simulink model "reto4_simu"  (R2024a)
settings: Solver=FixedStepAuto  StartTime=0.0  StopTime=20.0  FixedStep=0.0001  RelTol=1e-3
libraries: cstblocks x2, simulink x1
settings Model: Creator=Usuario  LastModifiedBy=Usuario

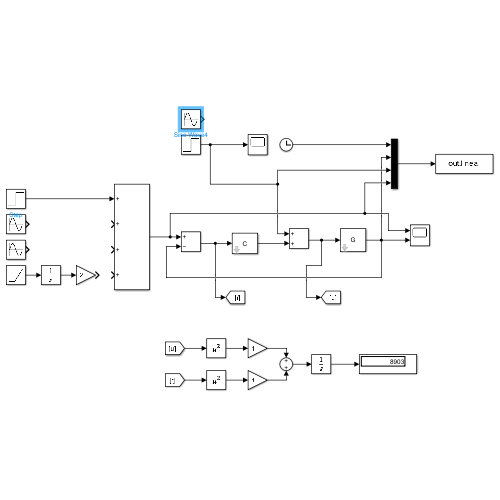
[thumbnail: Simulink's stored preview of the top-level diagram]
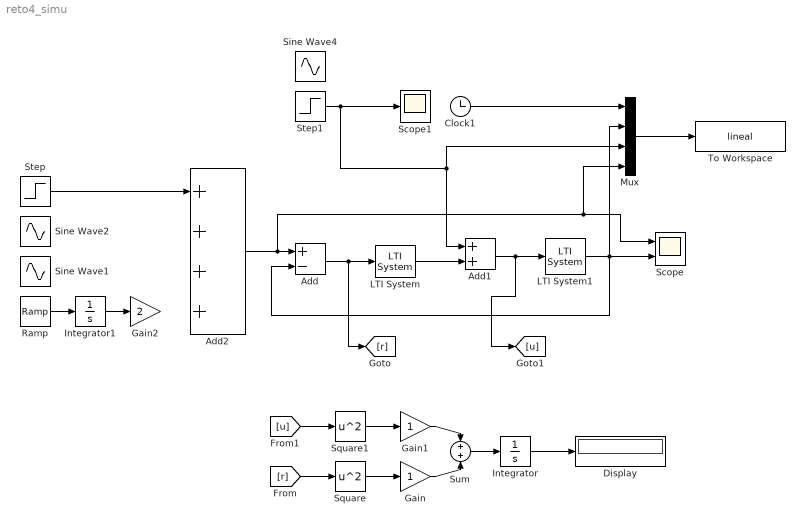
== system reto4_simu ==
  Add : Sum  Inputs=+-
  Add1 : Sum
  Add2 : Sum  Inputs=++++
  Clock1 : Clock
  Display : Display
  Gain : Gain
  Gain1 : Gain
  Gain2 : Gain  Gain=2
  Integrator : Integrator
  Integrator1 : Integrator
  LTI System : cstblocks/LTI System  sys=C  IC=[]  PadeOrder=0
  LTI System1 : cstblocks/LTI System  sys=G  IC=[]  PadeOrder=0
  Mux : Mux
  Ramp : simulink/Sources/Ramp  slope=1  start=0  InitialOutput=0
  Scope : Scope  NumInputPorts=2
  Scope1 : Scope
  Sine Wave1 : Sin  Frequency=2  Phase=pi/2+6  SampleTime=0
  Sine Wave2 : Sin  Frequency=2  SampleTime=0
  Sine Wave4 : Sin  Phase=pi  SampleTime=0
  Square : Math  Operator=square
  Square1 : Math  Operator=square
  Step : Step  Time=0  After=2  SampleTime=0
  Step1 : Step  Time=0  After=50  SampleTime=0
  Sum : Sum
  To Workspace : ToWorkspace  VariableName=lineal  SampleTime=-1
  wires:
  LTI System1/1 -> Mux/2, Scope/2, Add/2
  Add1/1 -> [u], LTI System1/1
  LTI System/1 -> Add1/2
  Add/1 -> [r], LTI System/1
  Add2/1 -> Mux/4, Scope/1, Add/1
  [r] -> Square/1
  [u] -> Square1/1
  Square/1 -> Gain/1
  Square1/1 -> Gain1/1
  Gain1/1 -> Sum/1
  Gain/1 -> Sum/2
  Sum/1 -> Integrator/1
  Integrator/1 -> Display/1
  Ramp/1 -> Integrator1/1
  Integrator1/1 -> Gain2/1
  Step/1 -> Add2/1
  Clock1/1 -> Mux/1
  Mux/1 -> To Workspace/1
  Step1/1 -> Scope1/1, Add1/1, Mux/3
